simulink model "DC_motor_statespace"  (R2015b)
settings: Solver=VariableStepAuto  StartTime=0.0  StopTime=10.0  RelTol=1e-3
undefined symbols (not defined in the file): A, B, C, x0
settings Model: Creator=mgreiff  LastModifiedBy=mgreiff

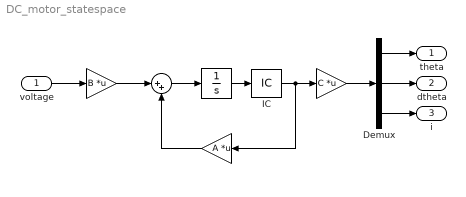
== system DC_motor_statespace ==
  voltage : Inport  PortDimensions=1
  " " : Sum  Inputs=|++
  "  " : Gain  Gain=B  Multiplication=Matrix(K*u)
  "   " : Integrator
  "    " : Gain  Gain=A  Multiplication=Matrix(K*u)
  "       " : Gain  Gain=C  Multiplication=Matrix(K*u)
  Demux : Demux  Outputs=3
  IC : InitialCondition  Value=x0
  theta : Outport  PortDimensions=1
  dtheta : Outport  Port=2  PortDimensions=1
  i : Outport  Port=3  PortDimensions=1
  wires:
  voltage/1 -> "  "/1
  " "/1 -> "   "/1
  "  "/1 -> " "/1
  "   "/1 -> IC/1
  "    "/1 -> " "/2
  "       "/1 -> Demux/1
  Demux/1 -> theta/1
  Demux/2 -> dtheta/1
  Demux/3 -> i/1
  IC/1 -> "    "/1, "       "/1
